simulink model "robotarm_pretrained"  (R2018b)
settings: Solver=FixedStepAuto  StartTime=0.0  StopTime=10  RelTol=1e-3  AbsTol=1e-6
undefined symbols (not defined in the file or in its folder): options
libraries: neural x132, simulink x2
(part 2 of 6)

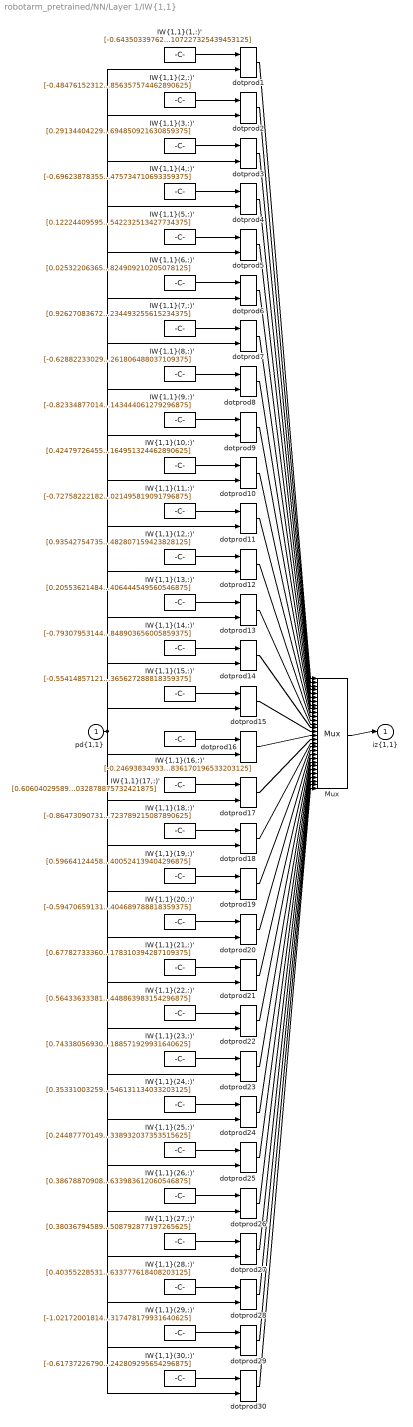
== system robotarm_pretrained/NN/Layer 1/IW{1,1} ==
  "pd{1,1}" : Inport  PortDimensions=10
      mask Display: e = 0.06;c1 = [120 230 180]/255;c2 = ([120 230 180]+0)/(256+128);c3 = ([120 230 180]+128)/(256+128);patch([0 1 1 0],[0 0 1 1],c1);patch([0 1 1 1-e 1-e 0+e],[0 0 1 1-e 0+e 0+e],c2);patch([0 0 1 1-e 0+e 0+e],[0 1 1 1-e 1-e 0+e],c3);plot([0 1 1 0 0],[0 0 1 1 0]);
  "IW{1,1}(1,:)'" : Constant  Value=[-0.64350339762783004271540221452596597373485565185546875;0.89913514336183941733082747305161319673061370849609375;-0.394377299783757795381688993074931204319000244140625;-0.73656593580094631423804685255163349211215972900390625;0.20561726214294895331846646513440646231174468994140625;-0.524044545421606056123664529877714812755584716796875;0.8311794536283019230182844694354571402072906494140625;0.72924618641789773487715820010635070502758026123046875;0.0100602920329538499111254878926047240383923053741455078125;0.55049304229430806589817848362145014107227325439453125]
      mask Display: e = 0.06;c1 = [120 150 230]/255;c2 = ([120 150 230]+0)/383;c3 = ([120 150 230]+128)/383;patch([0 1 1 0],[0 0 1 1],c1);patch([0 1 1 1-e 1-e 0+e],[0 0 1 1-e 0+e 0+e],c2);patch([0 0 1 1-e 0+e 0+e],[0 1 1 1-e 1-e 0+e],c3);plot([0 1 1 0 0],[0 0 1 1 0]);disp('Weights');
  "IW{1,1}(10,:)'" : Constant  Value=[0.4247972645502964272878898555063642561435699462890625;0.269860711531129060514189177411026321351528167724609375;0.339652704113527048601639535263529978692531585693359375;-0.7011806963928253200180051862844265997409820556640625;0.81999905126730399107515268042334355413913726806640625;-0.0981102413846167975552958750995458103716373443603515625;-0.8830937342912383858362090904847718775272369384765625;0.80695122982498190822298056446015834808349609375;-0.49958163471078920192525174570619128644466400146484375;0.713323465367589282237759107374586164951324462890625]
      mask Display: e = 0.06;c1 = [120 150 230]/255;c2 = ([120 150 230]+0)/383;c3 = ([120 150 230]+128)/383;patch([0 1 1 0],[0 0 1 1],c1);patch([0 1 1 1-e 1-e 0+e],[0 0 1 1-e 0+e 0+e],c2);patch([0 0 1 1-e 0+e 0+e],[0 1 1 1-e 1-e 0+e],c3);plot([0 1 1 0 0],[0 0 1 1 0]);disp('Weights');
  "IW{1,1}(11,:)'" : Constant  Value=[-0.72758222182049780979440356531995348632335662841796875;0.8149979182888886786173543441691435873508453369140625;0.94004901932021944777062572029535658657550811767578125;0.222298482599576130436247467514476738870143890380859375;-0.52537584741662168852371905813924968242645263671875;-0.67917660081824837714492559825885109603404998779296875;-0.129958873102197169924210129465791396796703338623046875;-0.1497066224255674538046179122829926200211048126220703125;-0.7821589950925946777005037802155129611492156982421875;-0.347580261909502030714946840816992335021495819091796875]
      mask Display: e = 0.06;c1 = [120 150 230]/255;c2 = ([120 150 230]+0)/383;c3 = ([120 150 230]+128)/383;patch([0 1 1 0],[0 0 1 1],c1);patch([0 1 1 1-e 1-e 0+e],[0 0 1 1-e 0+e 0+e],c2);patch([0 0 1 1-e 0+e 0+e],[0 1 1 1-e 1-e 0+e],c3);plot([0 1 1 0 0],[0 0 1 1 0]);disp('Weights');
  "IW{1,1}(12,:)'" : Constant  Value=[0.93542754735983602021320848507457412779331207275390625;0.04598685469958241345267424549092538654804229736328125;-0.06136820748890810250930627489651669748127460479736328125;-0.71265970414753276873653931033913977444171905517578125;0.4445330734346033541015685841557569801807403564453125;0.1453598052720599109743915278158965520560741424560546875;-0.321566135262894958746215934297651983797550201416015625;0.703664866384951626088195553165860474109649658203125;-1.1339440961807227825630661754985339939594268798828125;-0.59819193835228745559362550920923240482807159423828125]
      mask Display: e = 0.06;c1 = [120 150 230]/255;c2 = ([120 150 230]+0)/383;c3 = ([120 150 230]+128)/383;patch([0 1 1 0],[0 0 1 1],c1);patch([0 1 1 1-e 1-e 0+e],[0 0 1 1-e 0+e 0+e],c2);patch([0 0 1 1-e 0+e 0+e],[0 1 1 1-e 1-e 0+e],c3);plot([0 1 1 0 0],[0 0 1 1 0]);disp('Weights');
  "IW{1,1}(13,:)'" : Constant  Value=[0.205536214842288400550529559041024185717105865478515625;-0.65076279835128658657339428827981464564800262451171875;-0.54292056972558644378779035832849331200122833251953125;0.7360287358764046050652041230932809412479400634765625;0.198994359149927191321438613158534280955791473388671875;-0.07170276861816138325167457878706045448780059814453125;0.25418394334136917844801928367814980447292327880859375;0.229271648032539465678070200738147832453250885009765625;1.1636053825875929401689745645853690803050994873046875;0.8399344979335221506033803962054662406444549560546875]
      mask Display: e = 0.06;c1 = [120 150 230]/255;c2 = ([120 150 230]+0)/383;c3 = ([120 150 230]+128)/383;patch([0 1 1 0],[0 0 1 1],c1);patch([0 1 1 1-e 1-e 0+e],[0 0 1 1-e 0+e 0+e],c2);patch([0 0 1 1-e 0+e 0+e],[0 1 1 1-e 1-e 0+e],c3);plot([0 1 1 0 0],[0 0 1 1 0]);disp('Weights');
  "IW{1,1}(14,:)'" : Constant  Value=[-0.793079531446764907087754181702621281147003173828125;-0.425998786618885849630800066734082065522670745849609375;0.61972216508642763432845868010190315544605255126953125;-0.17227988464149091019095294541330076754093170166015625;0.7840827339085383318462163515505380928516387939453125;0.374321576511434328526917170165688730776309967041015625;-0.77066109725890530324221572300302796065807342529296875;-0.533432667390606685131615449790842831134796142578125;0.50371547567957841717856126706465147435665130615234375;-0.397107116539185511783216497860848903656005859375]
      mask Display: e = 0.06;c1 = [120 150 230]/255;c2 = ([120 150 230]+0)/383;c3 = ([120 150 230]+128)/383;patch([0 1 1 0],[0 0 1 1],c1);patch([0 1 1 1-e 1-e 0+e],[0 0 1 1-e 0+e 0+e],c2);patch([0 0 1 1-e 0+e 0+e],[0 1 1 1-e 1-e 0+e],c3);plot([0 1 1 0 0],[0 0 1 1 0]);disp('Weights');
  "IW{1,1}(15,:)'" : Constant  Value=[-0.55414857121611060808419324530404992401599884033203125;0.6816969884788803835107273698667995631694793701171875;-0.2769192349841465006221596922841854393482208251953125;0.51961818011582183718388705528923310339450836181640625;-0.255189976239418581105411476528388448059558868408203125;0.87559595332260775624177995268837548792362213134765625;0.58938436441075603422490303273661993443965911865234375;0.361652836539093580636716751541825942695140838623046875;0.84540457464287055433516115954262204468250274658203125;0.209564688022934431099741914295009337365627288818359375]
      mask Display: e = 0.06;c1 = [120 150 230]/255;c2 = ([120 150 230]+0)/383;c3 = ([120 150 230]+128)/383;patch([0 1 1 0],[0 0 1 1],c1);patch([0 1 1 1-e 1-e 0+e],[0 0 1 1-e 0+e 0+e],c2);patch([0 0 1 1-e 0+e 0+e],[0 1 1 1-e 1-e 0+e],c3);plot([0 1 1 0 0],[0 0 1 1 0]);disp('Weights');
  "IW{1,1}(16,:)'" : Constant  Value=[-0.246938349332889217624398270345409400761127471923828125;-0.438405413004595179149447403688100166618824005126953125;0.81830243710484984465125535280094482004642486572265625;-0.4728937076758945590171379080857150256633758544921875;0.033305214463347478093258047238123253919184207916259765625;1.2397309430933762808280107492464594542980194091796875;0.0999184542206135450914672446742770262062549591064453125;0.192742051896790111964463676486047916114330291748046875;-0.5670895899983252608222983326413668692111968994140625;-0.345446951066478658010083790941280312836170196533203125]
      mask Display: e = 0.06;c1 = [120 150 230]/255;c2 = ([120 150 230]+0)/383;c3 = ([120 150 230]+128)/383;patch([0 1 1 0],[0 0 1 1],c1);patch([0 1 1 1-e 1-e 0+e],[0 0 1 1-e 0+e 0+e],c2);patch([0 0 1 1-e 0+e 0+e],[0 1 1 1-e 1-e 0+e],c3);plot([0 1 1 0 0],[0 0 1 1 0]);disp('Weights');
  "IW{1,1}(17,:)'" : Constant  Value=[0.6060402958918249538555755862034857273101806640625;0.90527222388835648647642528885626234114170074462890625;0.12462405990060532179342089875717647373676300048828125;-0.126943651050287209525180287528201006352901458740234375;0.354053250721932555311610713033587671816349029541015625;1.003070002057440124332288178266026079654693603515625;-0.0060460349641447141966210665486869402229785919189453125;-0.870498324739053419563106217538006603717803955078125;0.226545437049204212431874339017667807638645172119140625;0.472153150642403651726652924480731599032878875732421875]
      mask Display: e = 0.06;c1 = [120 150 230]/255;c2 = ([120 150 230]+0)/383;c3 = ([120 150 230]+128)/383;patch([0 1 1 0],[0 0 1 1],c1);patch([0 1 1 1-e 1-e 0+e],[0 0 1 1-e 0+e 0+e],c2);patch([0 0 1 1-e 0+e 0+e],[0 1 1 1-e 1-e 0+e],c3);plot([0 1 1 0 0],[0 0 1 1 0]);disp('Weights');
  "IW{1,1}(18,:)'" : Constant  Value=[-0.86473090731057389302094406957621686160564422607421875;-0.85878435263240715524801771607599221169948577880859375;0.5589885033032706562750036027864553034305572509765625;-0.91530164106625877540324154324480332434177398681640625;0.76175383235007421145468242684728465974330902099609375;0.08369624509664556899490861496815341524779796600341796875;-0.3834092454451016873662183570559136569499969482421875;-0.5294959193616033399365505829337053000926971435546875;0.5345358981765062633684237880515865981578826904296875;0.166529697027367584727386429221951402723789215087890625]
      mask Display: e = 0.06;c1 = [120 150 230]/255;c2 = ([120 150 230]+0)/383;c3 = ([120 150 230]+128)/383;patch([0 1 1 0],[0 0 1 1],c1);patch([0 1 1 1-e 1-e 0+e],[0 0 1 1-e 0+e 0+e],c2);patch([0 0 1 1-e 0+e 0+e],[0 1 1 1-e 1-e 0+e],c3);plot([0 1 1 0 0],[0 0 1 1 0]);disp('Weights');
  "IW{1,1}(19,:)'" : Constant  Value=[0.596641244582879703983735453221015632152557373046875;-0.404749794363383152973057121926103718578815460205078125;-0.6200396131660228515869448528974317014217376708984375;0.77034399110490114903626590603380464017391204833984375;-0.16708966387306489753683536036987788975238800048828125;-0.478801908990822921996510785902501083910465240478515625;-0.912799998333343243217541385092772543430328369140625;0.9061719071483416154677570375497452914714813232421875;0.35448824018329927465487116933218203485012054443359375;0.313057634984507504594120064211892895400524139404296875]
      mask Display: e = 0.06;c1 = [120 150 230]/255;c2 = ([120 150 230]+0)/383;c3 = ([120 150 230]+128)/383;patch([0 1 1 0],[0 0 1 1],c1);patch([0 1 1 1-e 1-e 0+e],[0 0 1 1-e 0+e 0+e],c2);patch([0 0 1 1-e 0+e 0+e],[0 1 1 1-e 1-e 0+e],c3);plot([0 1 1 0 0],[0 0 1 1 0]);disp('Weights');
  "IW{1,1}(2,:)'" : Constant  Value=[-0.484761523128782123581714813553844578564167022705078125;0.9668077348744537058422565678483806550502777099609375;0.74093670068446471077550086192786693572998046875;0.227152637143275437647815806485596112906932830810546875;-0.19172605127726438656310392616433091461658477783203125;-0.1972512570044207269592817510783788748085498809814453125;0.54286777888365433941686433172435499727725982666015625;-0.362831808144802703264275578476372174918651580810546875;1.1302196168879270476992360272561199963092803955078125;0.76672029316854273250925189131521619856357574462890625]
      mask Display: e = 0.06;c1 = [120 150 230]/255;c2 = ([120 150 230]+0)/383;c3 = ([120 150 230]+128)/383;patch([0 1 1 0],[0 0 1 1],c1);patch([0 1 1 1-e 1-e 0+e],[0 0 1 1-e 0+e 0+e],c2);patch([0 0 1 1-e 0+e 0+e],[0 1 1 1-e 1-e 0+e],c3);plot([0 1 1 0 0],[0 0 1 1 0]);disp('Weights');
  "IW{1,1}(20,:)'" : Constant  Value=[-0.5947065913188371855113700803485698997974395751953125;0.88213037789516424158620111484196968376636505126953125;0.1789777728991974459216152126828092150390148162841796875;0.450386421751610754871109065788914449512958526611328125;-0.1380581067987025900567488179149222560226917266845703125;0.4583287360600205584404420733335427939891815185546875;-0.42618966788799406142373982220306061208248138427734375;-0.5171331281043383132356439091381616890430450439453125;-0.4881972428986596224120830811443738639354705810546875;-0.922796885587783943805106900981627404689788818359375]
      mask Display: e = 0.06;c1 = [120 150 230]/255;c2 = ([120 150 230]+0)/383;c3 = ([120 150 230]+128)/383;patch([0 1 1 0],[0 0 1 1],c1);patch([0 1 1 1-e 1-e 0+e],[0 0 1 1-e 0+e 0+e],c2);patch([0 0 1 1-e 0+e 0+e],[0 1 1 1-e 1-e 0+e],c3);plot([0 1 1 0 0],[0 0 1 1 0]);disp('Weights');
  "IW{1,1}(21,:)'" : Constant  Value=[0.677827333602184722849415265955030918121337890625;0.81581004978423854456792696510092355310916900634765625;0.006512024932718849141999317708950911764986813068389892578125;0.396807733680336560677659463181043975055217742919921875;0.79197000032309416983622440966428257524967193603515625;0.57680241787429842315049199896748177707195281982421875;-0.456502574791702253609315675930702127516269683837890625;0.00814435417052575792717927782859987928532063961029052734375;0.55983682431395609402358104489394463598728179931640625;-0.52274874341279475853383473804569803178310394287109375]
      mask Display: e = 0.06;c1 = [120 150 230]/255;c2 = ([120 150 230]+0)/383;c3 = ([120 150 230]+128)/383;patch([0 1 1 0],[0 0 1 1],c1);patch([0 1 1 1-e 1-e 0+e],[0 0 1 1-e 0+e 0+e],c2);patch([0 0 1 1-e 0+e 0+e],[0 1 1 1-e 1-e 0+e],c3);plot([0 1 1 0 0],[0 0 1 1 0]);disp('Weights');
  "IW{1,1}(22,:)'" : Constant  Value=[0.5643363338140632290418352567940019071102142333984375;-0.67616367898083151732890883067739196121692657470703125;-0.62730110306091690919316761210211552679538726806640625;-0.014287194868339299358428462483061593957245349884033203125;0.43535508425707314383856783024384640157222747802734375;1.2245443056280074234365429219906218349933624267578125;-0.57540092975733203584098873761831782758235931396484375;-0.252504107996767757082778871335904113948345184326171875;-0.053579030187962027598214120871489285491406917572021484375;0.68691656994514349587888091264176182448863983154296875]
      mask Display: e = 0.06;c1 = [120 150 230]/255;c2 = ([120 150 230]+0)/383;c3 = ([120 150 230]+128)/383;patch([0 1 1 0],[0 0 1 1],c1);patch([0 1 1 1-e 1-e 0+e],[0 0 1 1-e 0+e 0+e],c2);patch([0 0 1 1-e 0+e 0+e],[0 1 1 1-e 1-e 0+e],c3);plot([0 1 1 0 0],[0 0 1 1 0]);disp('Weights');
  "IW{1,1}(23,:)'" : Constant  Value=[0.743380569305817306968720004078932106494903564453125;0.409682982695028619080090948045835830271244049072265625;0.73971994550129693823947718556155450642108917236328125;0.69102301127528698021507125304196961224079132080078125;-0.8041831987411545146215985369053669273853302001953125;-0.285502226739036302216590001989970915019512176513671875;-0.309460080916341251366930009680800139904022216796875;0.73294375713257664539668212455580942332744598388671875;0.46254121737153985893797880635247565805912017822265625;0.11381188874253235499001135622165747918188571929931640625]
      mask Display: e = 0.06;c1 = [120 150 230]/255;c2 = ([120 150 230]+0)/383;c3 = ([120 150 230]+128)/383;patch([0 1 1 0],[0 0 1 1],c1);patch([0 1 1 1-e 1-e 0+e],[0 0 1 1-e 0+e 0+e],c2);patch([0 0 1 1-e 0+e 0+e],[0 1 1 1-e 1-e 0+e],c3);plot([0 1 1 0 0],[0 0 1 1 0]);disp('Weights');
  "IW{1,1}(24,:)'" : Constant  Value=[0.353310032598141920967549367560422979295253753662109375;0.2948525387154443677673043566755950450897216796875;-1.041573956454957983197573412326164543628692626953125;0.43092477489756964015299445236450992524623870849609375;0.95822665528707562376808937187888659536838531494140625;-0.62542038659245891007998352506547234952449798583984375;0.30791677935401595700426469193189404904842376708984375;-0.1677984237744238604772561984646017663180828094482421875;0.44852959912044554346977065506507642567157745361328125;-0.351906983948055807065458111537736840546131134033203125]
      mask Display: e = 0.06;c1 = [120 150 230]/255;c2 = ([120 150 230]+0)/383;c3 = ([120 150 230]+128)/383;patch([0 1 1 0],[0 0 1 1],c1);patch([0 1 1 1-e 1-e 0+e],[0 0 1 1-e 0+e 0+e],c2);patch([0 0 1 1-e 0+e 0+e],[0 1 1 1-e 1-e 0+e],c3);plot([0 1 1 0 0],[0 0 1 1 0]);disp('Weights');
  "IW{1,1}(25,:)'" : Constant  Value=[0.2448777014900244963779840645656804554164409637451171875;-0.50942228665457545133676831028424203395843505859375;1.1089062886981986277845635413541458547115325927734375;-0.8033419371532233288490942868520505726337432861328125;-0.1385737928625990489361896607078961096704006195068359375;0.452875545315557292980201964383013546466827392578125;-0.6629603131074193189675725079723633825778961181640625;-0.30911763968052430318067536063608713448047637939453125;-0.325631559256265357138460103669785894453525543212890625;0.432211732683116578446202993291080929338932037353515625]
      mask Display: e = 0.06;c1 = [120 150 230]/255;c2 = ([120 150 230]+0)/383;c3 = ([120 150 230]+128)/383;patch([0 1 1 0],[0 0 1 1],c1);patch([0 1 1 1-e 1-e 0+e],[0 0 1 1-e 0+e 0+e],c2);patch([0 0 1 1-e 0+e 0+e],[0 1 1 1-e 1-e 0+e],c3);plot([0 1 1 0 0],[0 0 1 1 0]);disp('Weights');
  "IW{1,1}(26,:)'" : Constant  Value=[0.386788709083743575956049198794062249362468719482421875;-0.06468667895265030332030420368027989752590656280517578125;-0.70356770999478335237853343642200343310832977294921875;-0.126660797414870185395585622245562262833118438720703125;-0.8177385055149051229506085292086936533451080322265625;-0.01165838477031644164483292769318723003380000591278076171875;-0.954195726609535999074296341859735548496246337890625;0.36342194829175944459365155125851742923259735107421875;-0.68605479404764146966755333778564818203449249267578125;0.354702698516822845231644123487058095633983612060546875]
      mask Display: e = 0.06;c1 = [120 150 230]/255;c2 = ([120 150 230]+0)/383;c3 = ([120 150 230]+128)/383;patch([0 1 1 0],[0 0 1 1],c1);patch([0 1 1 1-e 1-e 0+e],[0 0 1 1-e 0+e 0+e],c2);patch([0 0 1 1-e 0+e 0+e],[0 1 1 1-e 1-e 0+e],c3);plot([0 1 1 0 0],[0 0 1 1 0]);disp('Weights');
  "IW{1,1}(27,:)'" : Constant  Value=[0.38036794589249345310832950417534448206424713134765625;-0.55114535127494457267260941080166958272457122802734375;-0.61337214958270858122801882927888073027133941650390625;1.0635782930439676707834451008238829672336578369140625;-0.705828738089271379152478402829729020595550537109375;0.56613086192424100229203531853272579610347747802734375;0.245497172120174689258220723786507733166217803955078125;0.40187903006584324572258992702700197696685791015625;0.380104372538575374651514948709518648684024810791015625;-0.8424434576473720515110699125216342508792877197265625]
      mask Display: e = 0.06;c1 = [120 150 230]/255;c2 = ([120 150 230]+0)/383;c3 = ([120 150 230]+128)/383;patch([0 1 1 0],[0 0 1 1],c1);patch([0 1 1 1-e 1-e 0+e],[0 0 1 1-e 0+e 0+e],c2);patch([0 0 1 1-e 0+e 0+e],[0 1 1 1-e 1-e 0+e],c3);plot([0 1 1 0 0],[0 0 1 1 0]);disp('Weights');
  "IW{1,1}(28,:)'" : Constant  Value=[0.403552285319256964779555119093856774270534515380859375;-0.75232762799274632836699083782150410115718841552734375;-0.75225795062997480311395293028908781707286834716796875;0.692892899231679848526255227625370025634765625;0.782878242213735031640453598811291158199310302734375;0.07543684208847541150522175712467287667095661163330078125;-0.85187519065799843787090139812789857387542724609375;-0.401134491772782209029202249439549632370471954345703125;0.1980958370735229900905238764607929624617099761962890625;0.7728489294631242234601131713134236633777618408203125]
      mask Display: e = 0.06;c1 = [120 150 230]/255;c2 = ([120 150 230]+0)/383;c3 = ([120 150 230]+128)/383;patch([0 1 1 0],[0 0 1 1],c1);patch([0 1 1 1-e 1-e 0+e],[0 0 1 1-e 0+e 0+e],c2);patch([0 0 1 1-e 0+e 0+e],[0 1 1 1-e 1-e 0+e],c3);plot([0 1 1 0 0],[0 0 1 1 0]);disp('Weights');
  "IW{1,1}(29,:)'" : Constant  Value=[-1.0217200181492922528292410788708366453647613525390625;0.2954369405106345158884550983202643692493438720703125;-0.59855601845911665659372147274552844464778900146484375;0.001918239693158604701472835785125425900332629680633544921875;0.05605233948420100531517817898929934017360210418701171875;0.10041000466439446714428385121209430508315563201904296875;-0.98964428828395878401380514333141036331653594970703125;0.89570934466722429423413132099085487425327301025390625;0.461823465260232268736473315584589727222919464111328125;-0.31167217013115477985962797902175225317478179931640625]
      mask Display: e = 0.06;c1 = [120 150 230]/255;c2 = ([120 150 230]+0)/383;c3 = ([120 150 230]+128)/383;patch([0 1 1 0],[0 0 1 1],c1);patch([0 1 1 1-e 1-e 0+e],[0 0 1 1-e 0+e 0+e],c2);patch([0 0 1 1-e 0+e 0+e],[0 1 1 1-e 1-e 0+e],c3);plot([0 1 1 0 0],[0 0 1 1 0]);disp('Weights');
  "IW{1,1}(3,:)'" : Constant  Value=[0.2913440422950046571060056521673686802387237548828125;-0.9714008678358772019834077582345344126224517822265625;0.464372218362125721569100278429687023162841796875;0.8616984065803716674736278946511447429656982421875;-0.79252869791214519690214501679292879998683929443359375;-0.2420648524698242598507391676321276463568210601806640625;0.7787618472159414384492492899880744516849517822265625;0.33767490714051551226049241449800319969654083251953125;0.1683452760005501591678012118791230022907257080078125;0.006579559331508998652748854141236733994446694850921630859375]
      mask Display: e = 0.06;c1 = [120 150 230]/255;c2 = ([120 150 230]+0)/383;c3 = ([120 150 230]+128)/383;patch([0 1 1 0],[0 0 1 1],c1);patch([0 1 1 1-e 1-e 0+e],[0 0 1 1-e 0+e 0+e],c2);patch([0 0 1 1-e 0+e 0+e],[0 1 1 1-e 1-e 0+e],c3);plot([0 1 1 0 0],[0 0 1 1 0]);disp('Weights');
  "IW{1,1}(30,:)'" : Constant  Value=[-0.6173722679015252179368644647183828055858612060546875;0.91571182001431961072768217491102404892444610595703125;-0.07143619725956966426405614356553996913135051727294921875;-0.4865800246173253018611148945637978613376617431640625;0.1510144948899086181359763259024475701153278350830078125;-0.712602893049190111440793771180324256420135498046875;-0.2818625426286887059035279889940284192562103271484375;0.74096677278260758559014220736571587622165679931640625;-0.75687731540326252943629015135229565203189849853515625;-0.68112549043710035601151275841402821242809295654296875]
      mask Display: e = 0.06;c1 = [120 150 230]/255;c2 = ([120 150 230]+0)/383;c3 = ([120 150 230]+128)/383;patch([0 1 1 0],[0 0 1 1],c1);patch([0 1 1 1-e 1-e 0+e],[0 0 1 1-e 0+e 0+e],c2);patch([0 0 1 1-e 0+e 0+e],[0 1 1 1-e 1-e 0+e],c3);plot([0 1 1 0 0],[0 0 1 1 0]);disp('Weights');
  "IW{1,1}(4,:)'" : Constant  Value=[-0.696238783555175988482233151444233953952789306640625;0.6739915761771164692817137620295397937297821044921875;0.57953474440303853754130614106543362140655517578125;0.106395110573631324069054926440003328025341033935546875;-0.16302720588212460395283187608583830296993255615234375;-0.62368040895347032215312310654553584754467010498046875;-0.420990104285445754239702864651917479932308197021484375;0.027195183532918755509033559292220161296427249908447265625;-0.5488421924468391832618863190873526036739349365234375;-0.887110598959649276906702652922831475734710693359375]
      mask Display: e = 0.06;c1 = [120 150 230]/255;c2 = ([120 150 230]+0)/383;c3 = ([120 150 230]+128)/383;patch([0 1 1 0],[0 0 1 1],c1);patch([0 1 1 1-e 1-e 0+e],[0 0 1 1-e 0+e 0+e],c2);patch([0 0 1 1-e 0+e 0+e],[0 1 1 1-e 1-e 0+e],c3);plot([0 1 1 0 0],[0 0 1 1 0]);disp('Weights');
  "IW{1,1}(5,:)'" : Constant  Value=[0.1222440959538308724585675690832431428134441375732421875;0.11668208587122148867099014069026452489197254180908203125;-0.250471195244995337159110704305930994451045989990234375;0.32504151506372280788781381488661281764507293701171875;-0.0352315288523026293177053958061151206493377685546875;-0.5092983470438030568772092010476626455783843994140625;-1.0833441736960054413430043496191501617431640625;-0.9195448031288899759516652920865453779697418212890625;0.76865815838524353953431500485748983919620513916015625;-0.310474230356819924647737707346095703542232513427734375]
      mask Display: e = 0.06;c1 = [120 150 230]/255;c2 = ([120 150 230]+0)/383;c3 = ([120 150 230]+128)/383;patch([0 1 1 0],[0 0 1 1],c1);patch([0 1 1 1-e 1-e 0+e],[0 0 1 1-e 0+e 0+e],c2);patch([0 0 1 1-e 0+e 0+e],[0 1 1 1-e 1-e 0+e],c3);plot([0 1 1 0 0],[0 0 1 1 0]);disp('Weights');
  "IW{1,1}(6,:)'" : Constant  Value=[0.025322063656567854461609812233291449956595897674560546875;-0.84935802212492961249523659716942347586154937744140625;0.84691628007327246496771522288327105343341827392578125;0.2193907669725518871928215958178043365478515625;0.60007373045645173714746078985626809298992156982421875;0.5616112744494443642651049231062643229961395263671875;-0.86129383336074616384081537034944631159305572509765625;0.9785915122294055468188389568240381777286529541015625;-0.1824104172189261741099386426867567934095859527587890625;0.1349457361209190076056785301261697895824909210205078125]
      mask Display: e = 0.06;c1 = [120 150 230]/255;c2 = ([120 150 230]+0)/383;c3 = ([120 150 230]+128)/383;patch([0 1 1 0],[0 0 1 1],c1);patch([0 1 1 1-e 1-e 0+e],[0 0 1 1-e 0+e 0+e],c2);patch([0 0 1 1-e 0+e 0+e],[0 1 1 1-e 1-e 0+e],c3);plot([0 1 1 0 0],[0 0 1 1 0]);disp('Weights');
  "IW{1,1}(7,:)'" : Constant  Value=[0.926270836722067780755196508835069835186004638671875;0.046455665705923888941786259465516195632517337799072265625;-0.596200698570211518045880438876338303089141845703125;-0.09671600979068674386329718117849552072584629058837890625;0.03801088024033051626648926912821480073034763336181640625;0.11942466313379772324676508787888451479375362396240234375;-0.942573107937807463940771413035690784454345703125;0.1989070008255688637444080768545973114669322967529296875;-0.53499775274761762755559857396292500197887420654296875;-0.9693147794378571546758394106291234493255615234375]
      mask Display: e = 0.06;c1 = [120 150 230]/255;c2 = ([120 150 230]+0)/383;c3 = ([120 150 230]+128)/383;patch([0 1 1 0],[0 0 1 1],c1);patch([0 1 1 1-e 1-e 0+e],[0 0 1 1-e 0+e 0+e],c2);patch([0 0 1 1-e 0+e 0+e],[0 1 1 1-e 1-e 0+e],c3);plot([0 1 1 0 0],[0 0 1 1 0]);disp('Weights');
  "IW{1,1}(8,:)'" : Constant  Value=[-0.6288223302994839780666325168567709624767303466796875;-0.237233917748443712270045580225996673107147216796875;0.823073265718152757841608035960234701633453369140625;-0.29134596714094695979468951918534003198146820068359375;0.1223135869042724921396114723393111489713191986083984375;1.031226481216641399640820964123122394084930419921875;0.548304441350126570142720083822496235370635986328125;-1.141383833187413987531044767820276319980621337890625;0.01350949882905325659387951731105204089544713497161865234375;0.05896755613608072044140584466731525026261806488037109375]
      mask Display: e = 0.06;c1 = [120 150 230]/255;c2 = ([120 150 230]+0)/383;c3 = ([120 150 230]+128)/383;patch([0 1 1 0],[0 0 1 1],c1);patch([0 1 1 1-e 1-e 0+e],[0 0 1 1-e 0+e 0+e],c2);patch([0 0 1 1-e 0+e 0+e],[0 1 1 1-e 1-e 0+e],c3);plot([0 1 1 0 0],[0 0 1 1 0]);disp('Weights');
  "IW{1,1}(9,:)'" : Constant  Value=[-0.82334877014197882516555182519368827342987060546875;0.67189657200871211184534104177146218717098236083984375;-0.717891557737757590729188450495712459087371826171875;-0.04136931868725614303006210548119270242750644683837890625;0.88081210749973759543962614770862273871898651123046875;0.62723099610241617174466455253423191606998443603515625;0.1524878416895050492474439352008630521595478057861328125;-0.637370873623208655800453925621695816516876220703125;-0.2467734148758700951642452992018661461770534515380859375;0.52929466088057697259472433870541863143444061279296875]
      mask Display: e = 0.06;c1 = [120 150 230]/255;c2 = ([120 150 230]+0)/383;c3 = ([120 150 230]+128)/383;patch([0 1 1 0],[0 0 1 1],c1);patch([0 1 1 1-e 1-e 0+e],[0 0 1 1-e 0+e 0+e],c2);patch([0 0 1 1-e 0+e 0+e],[0 1 1 1-e 1-e 0+e],c3);plot([0 1 1 0 0],[0 0 1 1 0]);disp('Weights');
  Mux : Mux  Inputs=30
      mask Display: e = 0.06;c1 = [120 150 230]/255;c2 = ([120 150 230]+0)/383;c3 = ([120 150 230]+128)/383;patch([0 1 1 0],[0 0 1 1],c1);patch([0 1 1 1-e 1-e 0+e],[0 0 1 1-e 0+e 0+e],c2);patch([0 0 1 1-e 0+e 0+e],[0 1 1 1-e 1-e 0+e],c3);plot([0 1 1 0 0],[0 0 1 1 0]);disp('Mux');
  dotprod{1..30} (30 alike) : neural/Weight Functions/dotprod
  "iz{1,1}" : Outport
      mask Display: e = 0.06;c1 = [120 230 180]/255;c2 = ([120 230 180]+0)/(256+128);c3 = ([120 230 180]+128)/(256+128);patch([0 1 1 0],[0 0 1 1],c1);patch([0 1 1 1-e 1-e 0+e],[0 0 1 1-e 0+e 0+e],c2);patch([0 0 1 1-e 0+e 0+e],[0 1 1 1-e 1-e 0+e],c3);plot([0 1 1 0 0],[0 0 1 1 0]);
  wires:
  "IW{1,1}(1,:)'"/1 -> dotprod1/1
  "pd{1,1}"/1 -> dotprod1/2, dotprod2/2, dotprod3/2, dotprod4/2, dotprod5/2, dotprod6/2, dotprod7/2, dotprod8/2, dotprod9/2, dotprod10/2, dotprod11/2, dotprod12/2, dotprod13/2, dotprod14/2, dotprod15/2, dotprod16/2, dotprod17/2, dotprod18/2, dotprod19/2, dotprod20/2, dotprod21/2, dotprod22/2, dotprod23/2, dotprod24/2, dotprod25/2, dotprod26/2, dotprod27/2, dotprod28/2, dotprod29/2, dotprod30/2
  dotprod1/1 -> Mux/1
  "IW{1,1}(2,:)'"/1 -> dotprod2/1
  dotprod2/1 -> Mux/2
  "IW{1,1}(3,:)'"/1 -> dotprod3/1
  dotprod3/1 -> Mux/3
  "IW{1,1}(4,:)'"/1 -> dotprod4/1
  dotprod4/1 -> Mux/4
  "IW{1,1}(5,:)'"/1 -> dotprod5/1
  dotprod5/1 -> Mux/5
  "IW{1,1}(6,:)'"/1 -> dotprod6/1
  dotprod6/1 -> Mux/6
  "IW{1,1}(7,:)'"/1 -> dotprod7/1
  dotprod7/1 -> Mux/7
  "IW{1,1}(8,:)'"/1 -> dotprod8/1
  dotprod8/1 -> Mux/8
  "IW{1,1}(9,:)'"/1 -> dotprod9/1
  dotprod9/1 -> Mux/9
  "IW{1,1}(10,:)'"/1 -> dotprod10/1
  dotprod10/1 -> Mux/10
  "IW{1,1}(11,:)'"/1 -> dotprod11/1
  dotprod11/1 -> Mux/11
  "IW{1,1}(12,:)'"/1 -> dotprod12/1
  dotprod12/1 -> Mux/12
  "IW{1,1}(13,:)'"/1 -> dotprod13/1
  dotprod13/1 -> Mux/13
  "IW{1,1}(14,:)'"/1 -> dotprod14/1
  dotprod14/1 -> Mux/14
  "IW{1,1}(15,:)'"/1 -> dotprod15/1
  dotprod15/1 -> Mux/15
  "IW{1,1}(16,:)'"/1 -> dotprod16/1
  dotprod16/1 -> Mux/16
  "IW{1,1}(17,:)'"/1 -> dotprod17/1
  dotprod17/1 -> Mux/17
  "IW{1,1}(18,:)'"/1 -> dotprod18/1
  dotprod18/1 -> Mux/18
  "IW{1,1}(19,:)'"/1 -> dotprod19/1
  dotprod19/1 -> Mux/19
  "IW{1,1}(20,:)'"/1 -> dotprod20/1
  dotprod20/1 -> Mux/20
  "IW{1,1}(21,:)'"/1 -> dotprod21/1
  dotprod21/1 -> Mux/21
  "IW{1,1}(22,:)'"/1 -> dotprod22/1
  dotprod22/1 -> Mux/22
  "IW{1,1}(23,:)'"/1 -> dotprod23/1
  dotprod23/1 -> Mux/23
  "IW{1,1}(24,:)'"/1 -> dotprod24/1
  dotprod24/1 -> Mux/24
  "IW{1,1}(25,:)'"/1 -> dotprod25/1
  dotprod25/1 -> Mux/25
  "IW{1,1}(26,:)'"/1 -> dotprod26/1
  dotprod26/1 -> Mux/26
  "IW{1,1}(27,:)'"/1 -> dotprod27/1
  dotprod27/1 -> Mux/27
  "IW{1,1}(28,:)'"/1 -> dotprod28/1
  dotprod28/1 -> Mux/28
  "IW{1,1}(29,:)'"/1 -> dotprod29/1
  dotprod29/1 -> Mux/29
  "IW{1,1}(30,:)'"/1 -> dotprod30/1
  dotprod30/1 -> Mux/30
  Mux/1 -> "iz{1,1}"/1

== system robotarm_pretrained/NN/Layer 2/Delays 1 ==
  "p{2}" : Inport  PortDimensions=30
      mask Display: e = 0.06;c1 = [120 230 180]/255;c2 = ([120 230 180]+0)/(256+128);c3 = ([120 230 180]+128)/(256+128);patch([0 1 1 0],[0 0 1 1],c1);patch([0 1 1 1-e 1-e 0+e],[0 0 1 1-e 0+e 0+e],c2);patch([0 0 1 1-e 0+e 0+e],[0 1 1 1-e 1-e 0+e],c3);plot([0 1 1 0 0],[0 0 1 1 0]);
  mux : Mux  Inputs=1
      mask Display: e = 0.06;c1 = [120 150 230]/255;c2 = ([120 150 230]+0)/383;c3 = ([120 150 230]+128)/383;patch([0 1 1 0],[0 0 1 1],c1);patch([0 1 1 1-e 1-e 0+e],[0 0 1 1-e 0+e 0+e],c2);patch([0 0 1 1-e 0+e 0+e],[0 1 1 1-e 1-e 0+e],c3);plot([0 1 1 0 0],[0 0 1 1 0]);disp('Mux')
  "pd{2,1}" : Outport
      mask Display: e = 0.06;c1 = [120 230 180]/255;c2 = ([120 230 180]+0)/(256+128);c3 = ([120 230 180]+128)/(256+128);patch([0 1 1 0],[0 0 1 1],c1);patch([0 1 1 1-e 1-e 0+e],[0 0 1 1-e 0+e 0+e],c2);patch([0 0 1 1-e 0+e 0+e],[0 1 1 1-e 1-e 0+e],c3);plot([0 1 1 0 0],[0 0 1 1 0]);
  wires:
  "p{2}"/1 -> mux/1
  mux/1 -> "pd{2,1}"/1
